simulink model "assignment2_TwoChannel_FF_phri"  (R2021b)
settings: Solver=VariableStepAuto  StartTime=0.0  StopTime=10.0  RelTol=1e-3
undefined symbols (not defined in the file): A, Be, Bh, Bm, Bs, Dh, Dm, Ds, Fc, Flp, Jh, Ke, Km, Ks, Mm, Ms, Ph, TransportDelay, xe
libraries: simulink x2
settings Model: Creator=miche  LastModifiedBy=miche

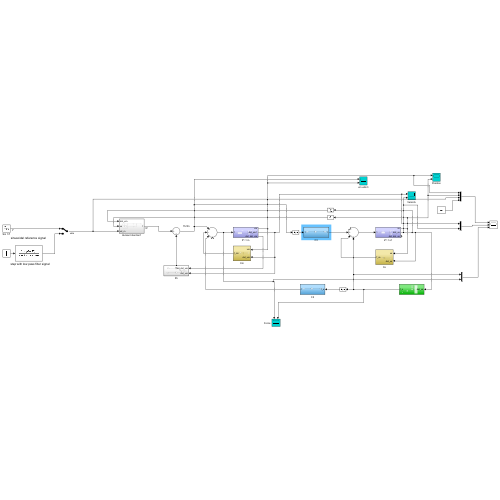
[thumbnail: Simulink's stored preview of the top-level diagram]
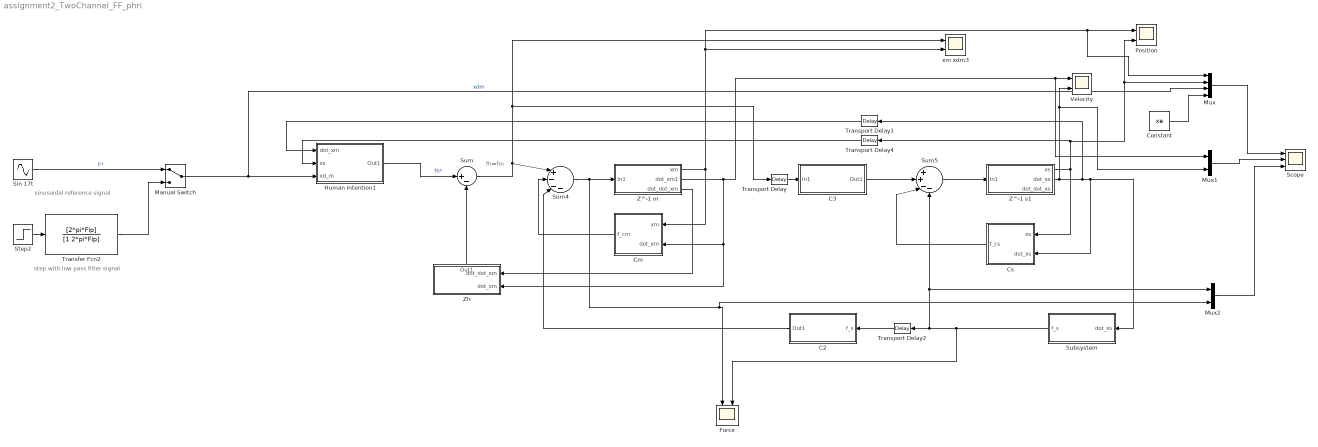
== system assignment2_TwoChannel_FF_phri ==
  note: fh=fm
  note: step with low pass filter signal
  note: sinusoidal reference signal
  C2 : Subsystem
  C3 : Subsystem
  Cm : Subsystem
  Constant : Constant  Value=xe
  Cs : Subsystem
  Force : Scope  NumInputPorts=2
  Human Intention1 : Subsystem
  Manual Switch : ManualSwitch
  Mux : Mux
  Mux1 : Mux  Inputs=2
  Mux2 : Mux  Inputs=2
  Position : Scope  NumInputPorts=2
  Scope : Scope  NumInputPorts=3
  Sin 17t : Sin  Amplitude=A  Frequency=2*pi*Fc  SampleTime=0
  Step2 : Step  Time=0.5  After=A  SampleTime=0
  Subsystem : Subsystem
  Sum : Sum  Inputs=|+-
  Sum4 : Sum  Inputs=|+---
  Sum5 : Sum  Inputs=|++--
  Transfer Fcn2 : TransferFcn  Numerator=[2*pi*Flp]  Denominator=[1 2*pi*Flp]
  Transport Delay{,1..2,4} (4 alike) : TransportDelay  DelayTime=TransportDelay
  Velocity : Scope  NumInputPorts=2
  Z^-1 m : Subsystem
  Z^-1 s1 : Subsystem
  Zh : Subsystem
      settings: PortSchema="{\"entries\":[{\"content\":{\"sides\":[{\"content\":{\"connectorIds\":[\"In1\",\"In2\"]},\"type\":\"ConnectorPlacement.EquallySpacedRectSide\",\"uuid\":\"a4a24afa-70f4-4279-8442-a10e90d1aef8\"},{\"content\":{\"connectorIds\":[],\"side\":\"RIGHT\"},\"type\":\"ConnectorPlacement.EquallySpacedRectSide\",\"uuid\":\"d7e1f09a-6379-4ac3-a140-38b478640de2\"},{\"content\":{\"connectorIds\":[\"Out1\"],\"side\":\"TOP\"},\"type\":\"ConnectorPlacement.EquallySpacedRectSide\",\"uuid\":\"ff61cea2-8b2e-45db-8140-b3346c095055\"}]},\"type\":\"ConnectorPlacement.EquallySpacedConnector\",\"uuid\":\"01c8eca0-3345-4aca-b450-750d9768d057\"}],\"packageUris\":[\"http://schema.mathworks.com/mf0/Connector/R2020b\"],\"version\":\"1.0\"}"
  xm xdm3 : Scope  NumInputPorts=2
  wires:
  Sum4/1 -> Mux2/2, Force/1, Z^-1 m/1(In1)
  Z^-1 m/1(xm) -> Cm/1(xm), Mux/1, Position/1, xm xdm3/2
  Step2/1 -> Transfer Fcn2/1
  C2/1(Out1) -> Sum4/3
  Z^-1 m/2(dot_xm1) -> Zh/2(dot_xm), Cm/2(dot_xm), Mux1/1, Velocity/1
  Sin 17t/1 -> Manual Switch/1  "F*"
  Transport Delay4/1 -> Human Intention1/2(xs)
  Cm/1(f_cm) -> Sum4/2
  Sum5/1 -> Z^-1 s1/1(In1)
  Subsystem/1(f_s) -> Force/2, Transport Delay2/1, Sum5/4, Mux2/1
  Cs/1(f_cs) -> Sum5/3
  Z^-1 s1/2(dot_xs) -> Mux1/2, Velocity/2, Transport Delay1/1, Subsystem/1(dot_xs), Cs/2(dot_xs)
  Transport Delay1/1 -> Human Intention1/1(dot_xm)
  Transport Delay2/1 -> C2/1(f_s)
  Manual Switch/1 -> Mux/3, Human Intention1/3(xd_m)  "xdm"
  Human Intention1/1(Out1) -> Sum/1  "fh*"
  Z^-1 s1/1(xs) -> Transport Delay4/1, Position/2, Mux/2, Cs/1(xs)
  Sum/1 -> Transport Delay/1, xm xdm3/1, Sum4/1
  Z^-1 m/3(dot_dot_xm) -> Zh/1(dot_dot_xm)
  Zh/1(Out1) -> Sum/2
  Transfer Fcn2/1 -> Manual Switch/2
  Transport Delay/1 -> C3/1(In1)
  C3/1(Out1) -> Sum5/2
  Constant/1 -> Mux/4
  Mux/1 -> Scope/1
  Mux1/1 -> Scope/2
  Mux2/1 -> Scope/3

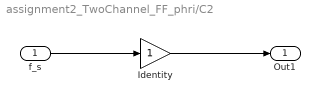
== system assignment2_TwoChannel_FF_phri/C2 ==
  f_s : Inport
  Identity : Gain
  Out1 : Outport
  wires:
  f_s/1 -> Identity/1
  Identity/1 -> Out1/1

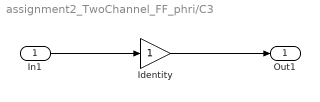
== system assignment2_TwoChannel_FF_phri/C3 ==
  In1 : Inport
  Identity : Gain
  Out1 : Outport
  wires:
  In1/1 -> Identity/1
  Identity/1 -> Out1/1

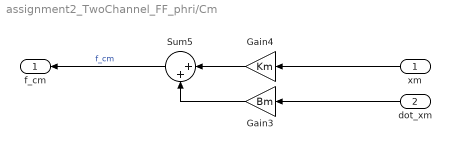
== system assignment2_TwoChannel_FF_phri/Cm ==
  xm : Inport
  dot_xm : Inport  Port=2
  Gain3 : Gain  Gain=Bm
  Gain4 : Gain  Gain=Km
  Sum5 : Sum  Inputs=|++
  f_cm : Outport
  wires:
  Gain4/1 -> Sum5/1
  Gain3/1 -> Sum5/2
  dot_xm/1 -> Gain3/1
  Sum5/1 -> f_cm/1  "f_cm"
  xm/1 -> Gain4/1

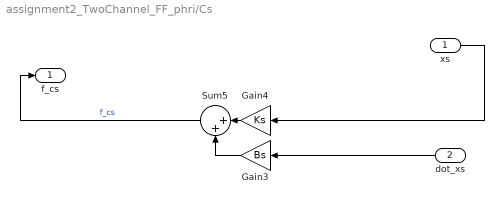
== system assignment2_TwoChannel_FF_phri/Cs ==
  xs : Inport
  dot_xs : Inport  Port=2
  Gain3 : Gain  Gain=Bs
  Gain4 : Gain  Gain=Ks
  Sum5 : Sum  Inputs=|++
  f_cs : Outport
  wires:
  Gain4/1 -> Sum5/1
  Gain3/1 -> Sum5/2
  dot_xs/1 -> Gain3/1
  Sum5/1 -> f_cs/1  "f_cs"
  xs/1 -> Gain4/1

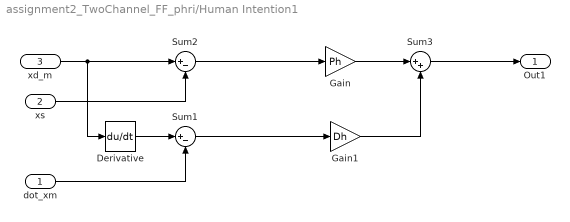
== system assignment2_TwoChannel_FF_phri/Human Intention1 ==
  dot_xm : Inport
  xs : Inport  Port=2
  xd_m : Inport  Port=3
  Derivative : Derivative
  Gain : Gain  Gain=Ph
  Gain1 : Gain  Gain=Dh
  Sum1 : Sum  Inputs=|+-
  Sum2 : Sum  Inputs=|+-
  Sum3 : Sum  Inputs=|++
  Out1 : Outport
  wires:
  xs/1 -> Sum2/2
  dot_xm/1 -> Sum1/2
  Sum2/1 -> Gain/1
  Sum1/1 -> Gain1/1
  Gain1/1 -> Sum3/2
  Gain/1 -> Sum3/1
  Sum3/1 -> Out1/1
  xd_m/1 -> Derivative/1, Sum2/1
  Derivative/1 -> Sum1/1

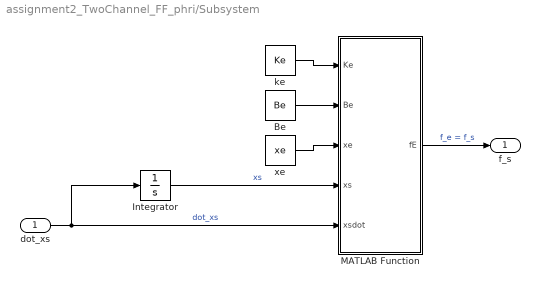
== system assignment2_TwoChannel_FF_phri/Subsystem ==
  dot_xs : Inport
  Be : Constant  Value=Be
  Integrator : Integrator
  MATLAB Function : MATLAB Function  TreatAsAtomicUnit=on
  ke : Constant  Value=Ke
  xe : Constant  Value=xe
  f_s : Outport
  wires:
  Integrator/1 -> MATLAB Function/4(xs)  "xs"
  MATLAB Function/1(fE) -> f_s/1  "f_e = f_s"
  dot_xs/1 -> Integrator/1, MATLAB Function/5(xsdot)  "dot_xs"
  ke/1 -> MATLAB Function/1(Ke)
  xe/1 -> MATLAB Function/3(xe)
  Be/1 -> MATLAB Function/2(Be)

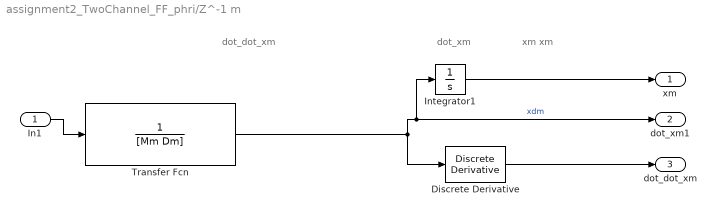
== system assignment2_TwoChannel_FF_phri/Z^-1 m ==
  note: dot_dot_xm
  note: dot_xm
  note: xm
      | xm
  In1 : Inport
  Discrete Derivative : simulink/Discrete/Discrete Derivative  gainval=1.0  ICPrevScaledInput=0.0  OutMin=[]  OutMax=[]  OutDataType=fixdt(1, 16)  OutScaling=2^-10  DoSatur=off
  Integrator1 : Integrator
  Transfer Fcn : TransferFcn  Denominator=[Mm Dm]
  xm : Outport
  dot_xm1 : Outport  Port=2
  dot_dot_xm : Outport  Port=3
  wires:
  Integrator1/1 -> xm/1
  Transfer Fcn/1 -> dot_xm1/1, Integrator1/1, Discrete Derivative/1  "xdm"
  In1/1 -> Transfer Fcn/1
  Discrete Derivative/1 -> dot_dot_xm/1

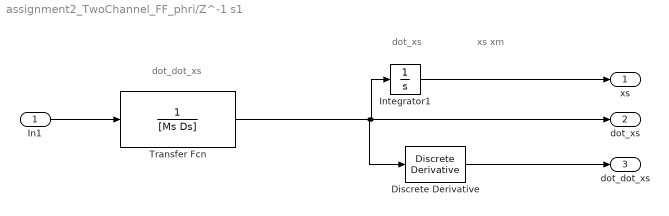
== system assignment2_TwoChannel_FF_phri/Z^-1 s1 ==
  note: dot_dot_xs
  note: dot_xs
  note: xs
      | xm
  In1 : Inport
  Discrete Derivative : simulink/Discrete/Discrete Derivative  gainval=1.0  ICPrevScaledInput=0.0  OutMin=[]  OutMax=[]  OutDataType=fixdt(1, 16)  OutScaling=2^-10  DoSatur=off
  Integrator1 : Integrator
  Transfer Fcn : TransferFcn  Denominator=[Ms Ds]
  xs : Outport
  dot_xs : Outport  Port=2
  dot_dot_xs : Outport  Port=3
  wires:
  Transfer Fcn/1 -> dot_xs/1, Integrator1/1, Discrete Derivative/1
  Integrator1/1 -> xs/1
  Discrete Derivative/1 -> dot_dot_xs/1
  In1/1 -> Transfer Fcn/1

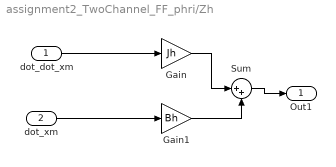
== system assignment2_TwoChannel_FF_phri/Zh ==
  dot_dot_xm : Inport
  dot_xm : Inport  Port=2
  Gain : Gain  Gain=Jh
  Gain1 : Gain  Gain=Bh
  Sum : Sum  Inputs=|++
  Out1 : Outport
  wires:
  Gain1/1 -> Sum/2
  Gain/1 -> Sum/1
  Sum/1 -> Out1/1
  dot_xm/1 -> Gain1/1
  dot_dot_xm/1 -> Gain/1

== matlab function assignment2_TwoChannel_FF_phri/Subsystem/MATLAB Function ==
  data: Ke input; fE output; Be input; xe input; xs input; xsdot input
function fE = environment(Ke, Be, xe, xs, xsdot)
    if xs > xe
        fE = Ke * (xs - xe) + Be * xsdot; % Plot both contributions Ke and Be
    else
        fE = 0;
    end
end
